simulink model "rotationCount"  (R2018a)
settings: Solver=ode45  StartTime=0.0  StopTime=10.0  RelTol=1e-3  EnableMultiTasking=on
PreLoadFcn:
  | load crankSpeedData
settings Model: Creator=jrivitus  LastModifiedBy=bneiswan
settings DataIOCC: ExternalInput=[t,crank_speed]  LimitDataPoints=on  LoadExternalInput=on  SaveFormat=Array
settings OptimizationCC: ExpressionDepthLimit=2147483647  LifeSpan=inf
settings DebuggingCC: UnderspecifiedInitializationDetection=Classic  MergeDetectMultiDrivingBlocksExec=none  MultiTaskDSMMsg=warning  MultiTaskCondExecSysMsg=none  ParameterPrecisionLossMsg=none  FcnCallInpInsideContextMsg=warning  AllowSymbolicDim=off  StateNameClashWarn=warning  SFUnexpectedBacktrackingDiag=warning  SFNoUnconditionalDefaultTransitionDiag=warning  SFExecutionAtInitializationDiag=none
settings HardwareCC: ProdBitPerPointer=32  ProdBitPerSizeT=32  ProdBitPerPtrDiffT=32  ProdLargestAtomicFloat=None  ProdIntDivRoundTo=Undefined  ProdEndianess=Unspecified  ProdWordSize=32  ProdHWDeviceType=32-bit Generic
settings ModelReferenceCC: PropagateSignalLabelsOutOfModel=off
settings CodeAppCC: StateflowObjectComments=on
settings GRTTargetCC: TargetLangStandard=C89/C90 (ANSI)  GeneratePreprocessorConditionals=Disable all  CombineOutputUpdateFcns=off  GRTInterface=on
settings ConfigComp: CovMetricSettings=dw  CovHtmlReporting=on  CovSaveCumulativeToWorkspaceVar=on  CovSaveSingleToWorkspaceVar=on  CovExternalEMLEnable=off  CovSFcnEnable=off

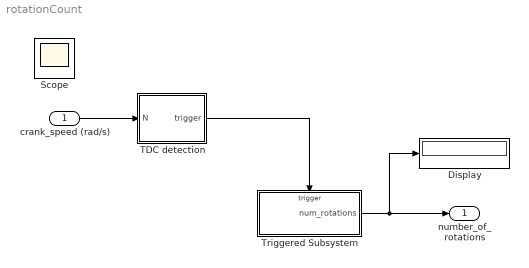
== system rotationCount ==
  crank_speed (rad/s) : Inport
  Display : Display
  TDC detection : Subsystem
  Triggered Subsystem : Subsystem  TreatAsAtomicUnit=on
  number_of_rotations : Outport
  Scope : Scope
  wires:
  TDC detection/1(trigger) -> Triggered Subsystem/Trigger
  Triggered Subsystem/1(num_rotations) -> number_of_rotations/1, Display/1
  crank_speed (rad/s)/1 -> TDC detection/1(N)

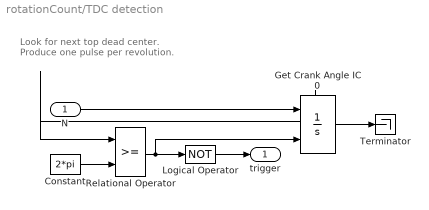
== system rotationCount/TDC detection ==
  note: Look for next top dead center.
      | Produce one pulse per revolution.
  N : Inport
  Constant : Constant  Value=2*pi
  Get Crank Angle IC 0 : Integrator  ExternalReset=rising  ShowStatePort=on
  Logical Operator : Logic  Operator=NOT  AllPortsSameDT=off  OutDataTypeStr=boolean
  Relational Operator : RelationalOperator  RndMeth=Nearest  InputSameDT=on
  Terminator : Terminator
  trigger : Outport  InitialOutput=0
  wires:
  N/1 -> Get Crank Angle IC 0/1
  Relational Operator/1 -> Logical Operator/1, Get Crank Angle IC 0/2
  Constant/1 -> Relational Operator/2
  Get Crank Angle IC 0/State -> Relational Operator/1
  Get Crank Angle IC 0/1 -> Terminator/1
  Logical Operator/1 -> trigger/1

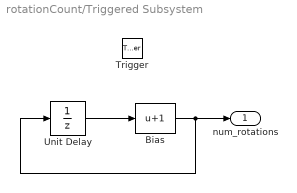
== system rotationCount/Triggered Subsystem ==
  Trigger : TriggerPort  VariantControl=Variant  PortDimensions=1
  Bias : Bias  Bias=1
  Unit Delay : UnitDelay  SampleTime=-1
  num_rotations : Outport
  wires:
  Unit Delay/1 -> Bias/1
  Bias/1 -> num_rotations/1, Unit Delay/1
